simulink model "chap14_12"  (Simulink 7.5)
settings: Solver=FixedStepDiscrete  StartTime=0.0  StopTime=0.0  RelTol=1e-3
undefined symbols (not defined in the file): gray, jet, strel
libraries: vipsnks x3, vipmorphops x2, vipconversions x1, vipsrcs x1
settings Model: Creator=yelinlin  LastModifiedBy=Administrator

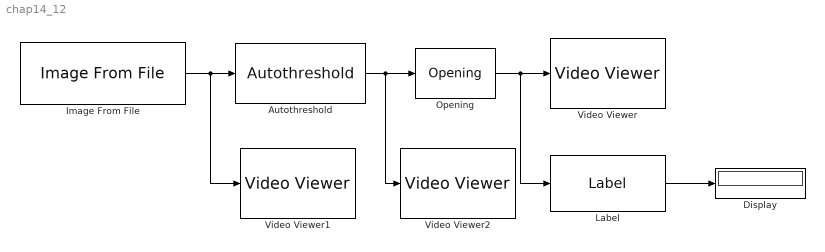
== system chap14_12 ==
  Autothreshold : vipconversions/Autothreshold  DialogController=vipDDGCreate  DialogControllerArgs=DataTag0  operator=>  threshOut=off  effMetricOut=off  userDefinedRange=off  umin=0  umax=255  outOfRngOpt=Warn and saturate  scaleThreshold=on  scaleFactor=0.9  P1Mode=Specify word length  P1WordLength=32  P1FracLength=30  P2Mode=Specify word length  P2WordLength=32  P2FracLength=22  P3Mode=Specify word length  P3WordLength=32  P3FracLength=14  P4Mode=Binary point scaling  P4WordLength=32  P4FracLength=15  Q1Mode=Specify word length  Q1WordLength=32  Q1FracLength=16  EMMode=Specify word length  EMWordLength=16  EMFracLength=14  roundingMode=Floor  overflowMode=off
  Display : Display
  Image From File : vipsrcs/Image From File  Tag=vipblks_nd  DialogController=vipDDGCreate  DialogControllerArgs=DataTag1  SystemSampleTime=-1  FileName=D:\Program Files\MATLAB\R2010a\toolbox\images\imdemos\coins.png  imagePorts=One multidimensional signal  Ts=inf  ImageDataType=Inherit from input image  Signed=on  WordLength=16  sdImageDataType=uint(8)  FractionLengthMode=User-defined  FractionLength=15  OutPortLabels=R|G|B
  Label : vipmorphops/Label  conn=8  output=Number of labels  outType=Automatic  lastLabel=maximum value of the output data type
  Opening : vipmorphops/Opening  nhoodsrc=Specify via dialog  strel=strel('disk',5)
  Video Viewer : vipsnks/Video Viewer  DialogControllerArgs=DataTag3  inputType=Obsolete7b  imagePorts=One multidimensional signal  useColorMap=off  colormapValue=gray(256)  specRange=off  minInputVal=0  maxInputVal=255  FigPos=[755 317 410 300]  AxisZoom=on  trueSizedOnce=off  OpenAtMdlStart=on
  Video Viewer1 : vipsnks/Video Viewer  DialogControllerArgs=DataTag5  inputType=Obsolete7b  imagePorts=One multidimensional signal  useColorMap=off  colormapValue=gray(256)  specRange=off  minInputVal=0  maxInputVal=255  FigPos=[755 317 410 300]  AxisZoom=on  trueSizedOnce=off  OpenAtMdlStart=on
  Video Viewer2 : vipsnks/Video Viewer  DialogControllerArgs=DataTag7  inputType=Obsolete7b  imagePorts=One multidimensional signal  useColorMap=off  colormapValue=jet(256)  specRange=off  minInputVal=0  maxInputVal=255  FigPos=[755 573 410 300]  AxisZoom=on  trueSizedOnce=off  OpenAtMdlStart=on
  wires:
  Image From File/1 -> Autothreshold/1, Video Viewer1/1
  Autothreshold/1 -> Opening/1, Video Viewer2/1
  Opening/1 -> Video Viewer/1, Label/1
  Label/1 -> Display/1
